simulink library "MBDS_Subsystems"  (R2018b)
settings: Solver=ode45  StartTime=0.0  StopTime=10.0  RelTol=1e-3
libraries: KIBES_Signal x1429, MBDS_Modules x44, simulink x2
(part 15 of 15)

== system MBDS_Subsystems/SUB_IoControl/PowerGroups ==
  bo_SendEnable : Inport
  in_DIAG_AnalogInputsPWR.IN_PWR_DIAG : KIBES_Signal/KIBES_Signal  MBDS_LibraryBlock=on  DatabaseKey=722  SignalName=DIAG_AnalogInputsPWR.IN_PWR_DIAG  SymbolName=DIAG_AnalogInputsPWR_IN_PWR_DIAG_000722  DataType=uint16  Init=1  Slope=1  Bias=0  DataSize=1  fpDataType=uint16  BlockIOType=Inport  DeviceType=0
  in_DIAG_AnalogInputsPWR.IN_PWR_G1_DIAG : KIBES_Signal/KIBES_Signal  MBDS_LibraryBlock=on  DatabaseKey=724  SignalName=DIAG_AnalogInputsPWR.IN_PWR_G1_DIAG  SymbolName=DIAG_AnalogInputsPWR_IN_PWR_G1_DIAG_000724  DataType=uint16  Init=1  Slope=1  Bias=0  DataSize=1  fpDataType=uint16  BlockIOType=Inport  DeviceType=0
  in_DIAG_AnalogInputsPWR.IN_PWR_G2_DIAG : KIBES_Signal/KIBES_Signal  MBDS_LibraryBlock=on  DatabaseKey=726  SignalName=DIAG_AnalogInputsPWR.IN_PWR_G2_DIAG  SymbolName=DIAG_AnalogInputsPWR_IN_PWR_G2_DIAG_000726  DataType=uint16  Init=1  Slope=1  Bias=0  DataSize=1  fpDataType=uint16  BlockIOType=Inport  DeviceType=0
  in_DIAG_AnalogInputsPWR.IN_PWR_G3_DIAG : KIBES_Signal/KIBES_Signal  MBDS_LibraryBlock=on  DatabaseKey=734  SignalName=DIAG_AnalogInputsPWR.IN_PWR_G3_DIAG  SymbolName=DIAG_AnalogInputsPWR_IN_PWR_G3_DIAG_000734  DataType=uint16  Init=1  Slope=1  Bias=0  DataSize=1  fpDataType=uint16  BlockIOType=Inport  DeviceType=0
  in_DIAG_AnalogInputsPWR.IN_PWR_G4_DIAG : KIBES_Signal/KIBES_Signal  MBDS_LibraryBlock=on  DatabaseKey=728  SignalName=DIAG_AnalogInputsPWR.IN_PWR_G4_DIAG  SymbolName=DIAG_AnalogInputsPWR_IN_PWR_G4_DIAG_000728  DataType=uint16  Init=1  Slope=1  Bias=0  DataSize=1  fpDataType=uint16  BlockIOType=Inport  DeviceType=0
  in_DIAG_AnalogInputsPWR.IN_PWR_G5_DIAG : KIBES_Signal/KIBES_Signal  MBDS_LibraryBlock=on  DatabaseKey=730  SignalName=DIAG_AnalogInputsPWR.IN_PWR_G5_DIAG  SymbolName=DIAG_AnalogInputsPWR_IN_PWR_G5_DIAG_000730  DataType=uint16  Init=1  Slope=1  Bias=0  DataSize=1  fpDataType=uint16  BlockIOType=Inport  DeviceType=0
  in_DIAG_AnalogInputsPWR.IN_PWR_G7_DIAG : KIBES_Signal/KIBES_Signal  MBDS_LibraryBlock=on  DatabaseKey=732  SignalName=DIAG_AnalogInputsPWR.IN_PWR_G7_DIAG  SymbolName=DIAG_AnalogInputsPWR_IN_PWR_G7_DIAG_000732  DataType=uint16  Init=1  Slope=1  Bias=0  DataSize=1  fpDataType=uint16  BlockIOType=Inport  DeviceType=0
  in_IN_AnalogInputsPWR.IN_PWR : KIBES_Signal/KIBES_Signal  MBDS_LibraryBlock=on  DatabaseKey=721  SignalName=IN_AnalogInputsPWR.IN_PWR  SymbolName=IN_AnalogInputsPWR_IN_PWR_000721  DataType=uint32  Init=0  Slope=1  Bias=0  DataSize=1  fpDataType=uint32  BlockIOType=Inport  DeviceType=0
  in_IN_AnalogInputsPWR.IN_PWR_G1 : KIBES_Signal/KIBES_Signal  MBDS_LibraryBlock=on  DatabaseKey=723  SignalName=IN_AnalogInputsPWR.IN_PWR_G1  SymbolName=IN_AnalogInputsPWR_IN_PWR_G1_000723  DataType=uint16  Init=0  Slope=1  Bias=0  DataSize=1  fpDataType=uint16  BlockIOType=Inport  DeviceType=0
  in_IN_AnalogInputsPWR.IN_PWR_G2 : KIBES_Signal/KIBES_Signal  MBDS_LibraryBlock=on  DatabaseKey=725  SignalName=IN_AnalogInputsPWR.IN_PWR_G2  SymbolName=IN_AnalogInputsPWR_IN_PWR_G2_000725  DataType=uint16  Init=0  Slope=1  Bias=0  DataSize=1  fpDataType=uint16  BlockIOType=Inport  DeviceType=0
  in_IN_AnalogInputsPWR.IN_PWR_G3 : KIBES_Signal/KIBES_Signal  MBDS_LibraryBlock=on  DatabaseKey=733  SignalName=IN_AnalogInputsPWR.IN_PWR_G3  SymbolName=IN_AnalogInputsPWR_IN_PWR_G3_000733  DataType=uint16  Init=0  Slope=1  Bias=0  DataSize=1  fpDataType=uint16  BlockIOType=Inport  DeviceType=0
  in_IN_AnalogInputsPWR.IN_PWR_G4 : KIBES_Signal/KIBES_Signal  MBDS_LibraryBlock=on  DatabaseKey=727  SignalName=IN_AnalogInputsPWR.IN_PWR_G4  SymbolName=IN_AnalogInputsPWR_IN_PWR_G4_000727  DataType=uint16  Init=0  Slope=1  Bias=0  DataSize=1  fpDataType=uint16  BlockIOType=Inport  DeviceType=0
  in_IN_AnalogInputsPWR.IN_PWR_G5 : KIBES_Signal/KIBES_Signal  MBDS_LibraryBlock=on  DatabaseKey=729  SignalName=IN_AnalogInputsPWR.IN_PWR_G5  SymbolName=IN_AnalogInputsPWR_IN_PWR_G5_000729  DataType=uint16  Init=0  Slope=1  Bias=0  DataSize=1  fpDataType=uint16  BlockIOType=Inport  DeviceType=0
  in_IN_AnalogInputsPWR.IN_PWR_G7 : KIBES_Signal/KIBES_Signal  MBDS_LibraryBlock=on  DatabaseKey=731  SignalName=IN_AnalogInputsPWR.IN_PWR_G7  SymbolName=IN_AnalogInputsPWR_IN_PWR_G7_000731  DataType=uint16  Init=0  Slope=1  Bias=0  DataSize=1  fpDataType=uint16  BlockIOType=Inport  DeviceType=0
  out_OUT_PCAN.Tx_Pwr.PWR_G1_Sts.MessageEnable : KIBES_Signal/KIBES_Signal  MBDS_LibraryBlock=on  DatabaseKey=1777  SignalName=OUT_PCAN.Tx_Pwr.PWR_G1_Sts.MessageEnable  SymbolName=OUT_PCAN_Tx_Pwr_PWR_G1_Sts_MessageEnable_001777  DataType=boolean  Init=0  Slope=1  Bias=0  DataSize=1  fpDataType=boolean  BlockIOType=Outport  DeviceType=0
  out_OUT_PCAN.Tx_Pwr.PWR_G1_Sts.PWR_Gx_DIAG : KIBES_Signal/KIBES_Signal  MBDS_LibraryBlock=on  DatabaseKey=1763  SignalName=OUT_PCAN.Tx_Pwr.PWR_G1_Sts.PWR_Gx_DIAG  SymbolName=OUT_PCAN_Tx_Pwr_PWR_G1_Sts_PWR_Gx_DIAG_001763  DataType=uint16  Init=0  Slope=1  Bias=0  DataSize=1  fpDataType=uint16  BlockIOType=Outport  DeviceType=0
  out_OUT_PCAN.Tx_Pwr.PWR_G1_Sts.PWR_Gx_Val : KIBES_Signal/KIBES_Signal  MBDS_LibraryBlock=on  DatabaseKey=1764  SignalName=OUT_PCAN.Tx_Pwr.PWR_G1_Sts.PWR_Gx_Val  SymbolName=OUT_PCAN_Tx_Pwr_PWR_G1_Sts_PWR_Gx_Val_001764  DataType=uint16  Init=0  Slope=1  Bias=0  DataSize=1  fpDataType=uint16  BlockIOType=Outport  DeviceType=0
  out_OUT_PCAN.Tx_Pwr.PWR_G2_Sts.MessageEnable : KIBES_Signal/KIBES_Signal  MBDS_LibraryBlock=on  DatabaseKey=1778  SignalName=OUT_PCAN.Tx_Pwr.PWR_G2_Sts.MessageEnable  SymbolName=OUT_PCAN_Tx_Pwr_PWR_G2_Sts_MessageEnable_001778  DataType=boolean  Init=0  Slope=1  Bias=0  DataSize=1  fpDataType=boolean  BlockIOType=Outport  DeviceType=0
  out_OUT_PCAN.Tx_Pwr.PWR_G2_Sts.PWR_Gx_DIAG : KIBES_Signal/KIBES_Signal  MBDS_LibraryBlock=on  DatabaseKey=1765  SignalName=OUT_PCAN.Tx_Pwr.PWR_G2_Sts.PWR_Gx_DIAG  SymbolName=OUT_PCAN_Tx_Pwr_PWR_G2_Sts_PWR_Gx_DIAG_001765  DataType=uint16  Init=0  Slope=1  Bias=0  DataSize=1  fpDataType=uint16  BlockIOType=Outport  DeviceType=0
  out_OUT_PCAN.Tx_Pwr.PWR_G2_Sts.PWR_Gx_Val : KIBES_Signal/KIBES_Signal  MBDS_LibraryBlock=on  DatabaseKey=1766  SignalName=OUT_PCAN.Tx_Pwr.PWR_G2_Sts.PWR_Gx_Val  SymbolName=OUT_PCAN_Tx_Pwr_PWR_G2_Sts_PWR_Gx_Val_001766  DataType=uint16  Init=0  Slope=1  Bias=0  DataSize=1  fpDataType=uint16  BlockIOType=Outport  DeviceType=0
  out_OUT_PCAN.Tx_Pwr.PWR_G3_Sts.MessageEnable : KIBES_Signal/KIBES_Signal  MBDS_LibraryBlock=on  DatabaseKey=1779  SignalName=OUT_PCAN.Tx_Pwr.PWR_G3_Sts.MessageEnable  SymbolName=OUT_PCAN_Tx_Pwr_PWR_G3_Sts_MessageEnable_001779  DataType=boolean  Init=0  Slope=1  Bias=0  DataSize=1  fpDataType=boolean  BlockIOType=Outport  DeviceType=0
  out_OUT_PCAN.Tx_Pwr.PWR_G3_Sts.PWR_Gx_DIAG : KIBES_Signal/KIBES_Signal  MBDS_LibraryBlock=on  DatabaseKey=1767  SignalName=OUT_PCAN.Tx_Pwr.PWR_G3_Sts.PWR_Gx_DIAG  SymbolName=OUT_PCAN_Tx_Pwr_PWR_G3_Sts_PWR_Gx_DIAG_001767  DataType=uint16  Init=0  Slope=1  Bias=0  DataSize=1  fpDataType=uint16  BlockIOType=Outport  DeviceType=0
  out_OUT_PCAN.Tx_Pwr.PWR_G3_Sts.PWR_Gx_Val : KIBES_Signal/KIBES_Signal  MBDS_LibraryBlock=on  DatabaseKey=1768  SignalName=OUT_PCAN.Tx_Pwr.PWR_G3_Sts.PWR_Gx_Val  SymbolName=OUT_PCAN_Tx_Pwr_PWR_G3_Sts_PWR_Gx_Val_001768  DataType=uint16  Init=0  Slope=1  Bias=0  DataSize=1  fpDataType=uint16  BlockIOType=Outport  DeviceType=0
  out_OUT_PCAN.Tx_Pwr.PWR_G4_Sts.MessageEnable : KIBES_Signal/KIBES_Signal  MBDS_LibraryBlock=on  DatabaseKey=1780  SignalName=OUT_PCAN.Tx_Pwr.PWR_G4_Sts.MessageEnable  SymbolName=OUT_PCAN_Tx_Pwr_PWR_G4_Sts_MessageEnable_001780  DataType=boolean  Init=0  Slope=1  Bias=0  DataSize=1  fpDataType=boolean  BlockIOType=Outport  DeviceType=0
  out_OUT_PCAN.Tx_Pwr.PWR_G4_Sts.PWR_Gx_DIAG : KIBES_Signal/KIBES_Signal  MBDS_LibraryBlock=on  DatabaseKey=1769  SignalName=OUT_PCAN.Tx_Pwr.PWR_G4_Sts.PWR_Gx_DIAG  SymbolName=OUT_PCAN_Tx_Pwr_PWR_G4_Sts_PWR_Gx_DIAG_001769  DataType=uint16  Init=0  Slope=1  Bias=0  DataSize=1  fpDataType=uint16  BlockIOType=Outport  DeviceType=0
  out_OUT_PCAN.Tx_Pwr.PWR_G4_Sts.PWR_Gx_Val : KIBES_Signal/KIBES_Signal  MBDS_LibraryBlock=on  DatabaseKey=1770  SignalName=OUT_PCAN.Tx_Pwr.PWR_G4_Sts.PWR_Gx_Val  SymbolName=OUT_PCAN_Tx_Pwr_PWR_G4_Sts_PWR_Gx_Val_001770  DataType=uint16  Init=0  Slope=1  Bias=0  DataSize=1  fpDataType=uint16  BlockIOType=Outport  DeviceType=0
  out_OUT_PCAN.Tx_Pwr.PWR_G5_Sts.MessageEnable : KIBES_Signal/KIBES_Signal  MBDS_LibraryBlock=on  DatabaseKey=1781  SignalName=OUT_PCAN.Tx_Pwr.PWR_G5_Sts.MessageEnable  SymbolName=OUT_PCAN_Tx_Pwr_PWR_G5_Sts_MessageEnable_001781  DataType=boolean  Init=0  Slope=1  Bias=0  DataSize=1  fpDataType=boolean  BlockIOType=Outport  DeviceType=0
  out_OUT_PCAN.Tx_Pwr.PWR_G5_Sts.PWR_Gx_DIAG : KIBES_Signal/KIBES_Signal  MBDS_LibraryBlock=on  DatabaseKey=1771  SignalName=OUT_PCAN.Tx_Pwr.PWR_G5_Sts.PWR_Gx_DIAG  SymbolName=OUT_PCAN_Tx_Pwr_PWR_G5_Sts_PWR_Gx_DIAG_001771  DataType=uint16  Init=0  Slope=1  Bias=0  DataSize=1  fpDataType=uint16  BlockIOType=Outport  DeviceType=0
  out_OUT_PCAN.Tx_Pwr.PWR_G5_Sts.PWR_Gx_Val : KIBES_Signal/KIBES_Signal  MBDS_LibraryBlock=on  DatabaseKey=1772  SignalName=OUT_PCAN.Tx_Pwr.PWR_G5_Sts.PWR_Gx_Val  SymbolName=OUT_PCAN_Tx_Pwr_PWR_G5_Sts_PWR_Gx_Val_001772  DataType=uint16  Init=0  Slope=1  Bias=0  DataSize=1  fpDataType=uint16  BlockIOType=Outport  DeviceType=0
  out_OUT_PCAN.Tx_Pwr.PWR_G7_Sts.MessageEnable : KIBES_Signal/KIBES_Signal  MBDS_LibraryBlock=on  DatabaseKey=1782  SignalName=OUT_PCAN.Tx_Pwr.PWR_G7_Sts.MessageEnable  SymbolName=OUT_PCAN_Tx_Pwr_PWR_G7_Sts_MessageEnable_001782  DataType=boolean  Init=0  Slope=1  Bias=0  DataSize=1  fpDataType=boolean  BlockIOType=Outport  DeviceType=0
  out_OUT_PCAN.Tx_Pwr.PWR_G7_Sts.PWR_Gx_DIAG : KIBES_Signal/KIBES_Signal  MBDS_LibraryBlock=on  DatabaseKey=1773  SignalName=OUT_PCAN.Tx_Pwr.PWR_G7_Sts.PWR_Gx_DIAG  SymbolName=OUT_PCAN_Tx_Pwr_PWR_G7_Sts_PWR_Gx_DIAG_001773  DataType=uint16  Init=0  Slope=1  Bias=0  DataSize=1  fpDataType=uint16  BlockIOType=Outport  DeviceType=0
  out_OUT_PCAN.Tx_Pwr.PWR_G7_Sts.PWR_Gx_Val : KIBES_Signal/KIBES_Signal  MBDS_LibraryBlock=on  DatabaseKey=1774  SignalName=OUT_PCAN.Tx_Pwr.PWR_G7_Sts.PWR_Gx_Val  SymbolName=OUT_PCAN_Tx_Pwr_PWR_G7_Sts_PWR_Gx_Val_001774  DataType=uint16  Init=0  Slope=1  Bias=0  DataSize=1  fpDataType=uint16  BlockIOType=Outport  DeviceType=0
  out_OUT_PCAN.Tx_Pwr.PWR_Sts.MessageEnable : KIBES_Signal/KIBES_Signal  MBDS_LibraryBlock=on  DatabaseKey=1783  SignalName=OUT_PCAN.Tx_Pwr.PWR_Sts.MessageEnable  SymbolName=OUT_PCAN_Tx_Pwr_PWR_Sts_MessageEnable_001783  DataType=boolean  Init=0  Slope=1  Bias=0  DataSize=1  fpDataType=boolean  BlockIOType=Outport  DeviceType=0
  out_OUT_PCAN.Tx_Pwr.PWR_Sts.PWR_DIAG : KIBES_Signal/KIBES_Signal  MBDS_LibraryBlock=on  DatabaseKey=1775  SignalName=OUT_PCAN.Tx_Pwr.PWR_Sts.PWR_DIAG  SymbolName=OUT_PCAN_Tx_Pwr_PWR_Sts_PWR_DIAG_001775  DataType=uint16  Init=0  Slope=1  Bias=0  DataSize=1  fpDataType=uint16  BlockIOType=Outport  DeviceType=0
  out_OUT_PCAN.Tx_Pwr.PWR_Sts.PWR_Val : KIBES_Signal/KIBES_Signal  MBDS_LibraryBlock=on  DatabaseKey=1776  SignalName=OUT_PCAN.Tx_Pwr.PWR_Sts.PWR_Val  SymbolName=OUT_PCAN_Tx_Pwr_PWR_Sts_PWR_Val_001776  DataType=uint32  Init=0  Slope=1  Bias=0  DataSize=1  fpDataType=uint32  BlockIOType=Outport  DeviceType=0
  wires:
  in_DIAG_AnalogInputsPWR.IN_PWR_G3_DIAG/1 -> out_OUT_PCAN.Tx_Pwr.PWR_G3_Sts.PWR_Gx_DIAG/1
  in_DIAG_AnalogInputsPWR.IN_PWR_G4_DIAG/1 -> out_OUT_PCAN.Tx_Pwr.PWR_G4_Sts.PWR_Gx_DIAG/1
  in_IN_AnalogInputsPWR.IN_PWR_G7/1 -> out_OUT_PCAN.Tx_Pwr.PWR_G7_Sts.PWR_Gx_Val/1
  in_IN_AnalogInputsPWR.IN_PWR_G3/1 -> out_OUT_PCAN.Tx_Pwr.PWR_G3_Sts.PWR_Gx_Val/1
  in_DIAG_AnalogInputsPWR.IN_PWR_G7_DIAG/1 -> out_OUT_PCAN.Tx_Pwr.PWR_G7_Sts.PWR_Gx_DIAG/1
  in_DIAG_AnalogInputsPWR.IN_PWR_G5_DIAG/1 -> out_OUT_PCAN.Tx_Pwr.PWR_G5_Sts.PWR_Gx_DIAG/1
  in_DIAG_AnalogInputsPWR.IN_PWR_G2_DIAG/1 -> out_OUT_PCAN.Tx_Pwr.PWR_G2_Sts.PWR_Gx_DIAG/1
  in_IN_AnalogInputsPWR.IN_PWR/1 -> out_OUT_PCAN.Tx_Pwr.PWR_Sts.PWR_Val/1
  in_DIAG_AnalogInputsPWR.IN_PWR_DIAG/1 -> out_OUT_PCAN.Tx_Pwr.PWR_Sts.PWR_DIAG/1
  in_DIAG_AnalogInputsPWR.IN_PWR_G1_DIAG/1 -> out_OUT_PCAN.Tx_Pwr.PWR_G1_Sts.PWR_Gx_DIAG/1
  in_IN_AnalogInputsPWR.IN_PWR_G4/1 -> out_OUT_PCAN.Tx_Pwr.PWR_G4_Sts.PWR_Gx_Val/1
  bo_SendEnable/1 -> out_OUT_PCAN.Tx_Pwr.PWR_G7_Sts.MessageEnable/1, out_OUT_PCAN.Tx_Pwr.PWR_Sts.MessageEnable/1, out_OUT_PCAN.Tx_Pwr.PWR_G5_Sts.MessageEnable/1, out_OUT_PCAN.Tx_Pwr.PWR_G4_Sts.MessageEnable/1, out_OUT_PCAN.Tx_Pwr.PWR_G3_Sts.MessageEnable/1, out_OUT_PCAN.Tx_Pwr.PWR_G2_Sts.MessageEnable/1, out_OUT_PCAN.Tx_Pwr.PWR_G1_Sts.MessageEnable/1
  in_IN_AnalogInputsPWR.IN_PWR_G5/1 -> out_OUT_PCAN.Tx_Pwr.PWR_G5_Sts.PWR_Gx_Val/1
  in_IN_AnalogInputsPWR.IN_PWR_G1/1 -> out_OUT_PCAN.Tx_Pwr.PWR_G1_Sts.PWR_Gx_Val/1
  in_IN_AnalogInputsPWR.IN_PWR_G2/1 -> out_OUT_PCAN.Tx_Pwr.PWR_G2_Sts.PWR_Gx_Val/1

== system MBDS_Subsystems/SUB_LinControl/AND1 ==
  note: AND
  u1 : Inport
  DataType : DataTypeConversion
  Operator : simulink/Logic and Bit Operations/Bitwise Operator  logicop=AND  UseBitMask=on  BitMask='FF'  BitMaskRealWorld=Stored Integer
  y : Outport
  wires:
  DataType/1 -> y/1
  u1/1 -> Operator/1
  Operator/1 -> DataType/1

== system MBDS_Subsystems/SUB_LinControl/AND2 ==
  note: AND
  u1 : Inport
  DataType : DataTypeConversion
  Operator : simulink/Logic and Bit Operations/Bitwise Operator  logicop=AND  UseBitMask=on  BitMask='FF00'  BitMaskRealWorld=Stored Integer
  y : Outport
  wires:
  DataType/1 -> y/1
  u1/1 -> Operator/1
  Operator/1 -> DataType/1

== system MBDS_Subsystems/SUB_SystemStates/NOT ==
  note: NOT
  u1 : Inport  OutDataTypeStr=boolean
  DataType : DataTypeConversion  OutDataTypeStr=boolean
  Operator : Logic  Operator=NOT  Inputs=1  AllPortsSameDT=off  OutDataTypeStr=boolean
  y : Outport
  wires:
  DataType/1 -> y/1
  u1/1 -> Operator/1
  Operator/1 -> DataType/1

== system MBDS_Subsystems/SUB_SystemStates/OR ==
  note: OR
  u1 : Inport  OutDataTypeStr=boolean
  u2 : Inport  Port=2  OutDataTypeStr=boolean
  u3 : Inport  Port=3  OutDataTypeStr=boolean
  u4 : Inport  Port=4  OutDataTypeStr=boolean
  u5 : Inport  Port=5  OutDataTypeStr=boolean
  u6 : Inport  Port=6  OutDataTypeStr=boolean
  u7 : Inport  Port=7  OutDataTypeStr=boolean
  u8 : Inport  Port=8  OutDataTypeStr=boolean
  DataType : DataTypeConversion  OutDataTypeStr=boolean
  Operator : Logic  Operator=OR  Inputs=8  AllPortsSameDT=off  OutDataTypeStr=boolean
  y : Outport
  wires:
  u8/1 -> Operator/8
  u7/1 -> Operator/7
  u6/1 -> Operator/6
  u5/1 -> Operator/5
  u4/1 -> Operator/4
  u3/1 -> Operator/3
  DataType/1 -> y/1
  u2/1 -> Operator/2
  u1/1 -> Operator/1
  Operator/1 -> DataType/1

== system MBDS_Subsystems/SUB_ExpIOControl/Outputs/AND ==
  note: AND
  u1 : Inport  OutDataTypeStr=boolean
  u2 : Inport  Port=2  OutDataTypeStr=boolean
  DataType : DataTypeConversion  OutDataTypeStr=boolean
  Operator : Logic  AllPortsSameDT=off  OutDataTypeStr=boolean
  y : Outport
  wires:
  DataType/1 -> y/1
  u2/1 -> Operator/2
  u1/1 -> Operator/1
  Operator/1 -> DataType/1

== system MBDS_Subsystems/SUB_ExpIOControl/Outputs/AND1 ==
  note: AND
  u1 : Inport  OutDataTypeStr=boolean
  u2 : Inport  Port=2  OutDataTypeStr=boolean
  DataType : DataTypeConversion  OutDataTypeStr=boolean
  Operator : Logic  AllPortsSameDT=off  OutDataTypeStr=boolean
  y : Outport
  wires:
  DataType/1 -> y/1
  u2/1 -> Operator/2
  u1/1 -> Operator/1
  Operator/1 -> DataType/1

== system MBDS_Subsystems/SUB_ExpIOControl/Outputs/AND10 ==
  note: AND
  u1 : Inport  OutDataTypeStr=boolean
  u2 : Inport  Port=2  OutDataTypeStr=boolean
  DataType : DataTypeConversion  OutDataTypeStr=boolean
  Operator : Logic  AllPortsSameDT=off  OutDataTypeStr=boolean
  y : Outport
  wires:
  DataType/1 -> y/1
  u2/1 -> Operator/2
  u1/1 -> Operator/1
  Operator/1 -> DataType/1

== system MBDS_Subsystems/SUB_ExpIOControl/Outputs/AND11 ==
  note: AND
  u1 : Inport  OutDataTypeStr=boolean
  u2 : Inport  Port=2  OutDataTypeStr=boolean
  DataType : DataTypeConversion  OutDataTypeStr=boolean
  Operator : Logic  AllPortsSameDT=off  OutDataTypeStr=boolean
  y : Outport
  wires:
  DataType/1 -> y/1
  u2/1 -> Operator/2
  u1/1 -> Operator/1
  Operator/1 -> DataType/1

== system MBDS_Subsystems/SUB_ExpIOControl/Outputs/AND12 ==
  note: AND
  u1 : Inport  OutDataTypeStr=boolean
  u2 : Inport  Port=2  OutDataTypeStr=boolean
  DataType : DataTypeConversion  OutDataTypeStr=boolean
  Operator : Logic  AllPortsSameDT=off  OutDataTypeStr=boolean
  y : Outport
  wires:
  DataType/1 -> y/1
  u2/1 -> Operator/2
  u1/1 -> Operator/1
  Operator/1 -> DataType/1

== system MBDS_Subsystems/SUB_ExpIOControl/Outputs/AND13 ==
  note: AND
  u1 : Inport  OutDataTypeStr=boolean
  u2 : Inport  Port=2  OutDataTypeStr=boolean
  DataType : DataTypeConversion  OutDataTypeStr=boolean
  Operator : Logic  AllPortsSameDT=off  OutDataTypeStr=boolean
  y : Outport
  wires:
  DataType/1 -> y/1
  u2/1 -> Operator/2
  u1/1 -> Operator/1
  Operator/1 -> DataType/1

== system MBDS_Subsystems/SUB_ExpIOControl/Outputs/AND14 ==
  note: AND
  u1 : Inport  OutDataTypeStr=boolean
  u2 : Inport  Port=2  OutDataTypeStr=boolean
  DataType : DataTypeConversion  OutDataTypeStr=boolean
  Operator : Logic  AllPortsSameDT=off  OutDataTypeStr=boolean
  y : Outport
  wires:
  DataType/1 -> y/1
  u2/1 -> Operator/2
  u1/1 -> Operator/1
  Operator/1 -> DataType/1

== system MBDS_Subsystems/SUB_ExpIOControl/Outputs/AND15 ==
  note: AND
  u1 : Inport  OutDataTypeStr=boolean
  u2 : Inport  Port=2  OutDataTypeStr=boolean
  DataType : DataTypeConversion  OutDataTypeStr=boolean
  Operator : Logic  AllPortsSameDT=off  OutDataTypeStr=boolean
  y : Outport
  wires:
  DataType/1 -> y/1
  u2/1 -> Operator/2
  u1/1 -> Operator/1
  Operator/1 -> DataType/1

== system MBDS_Subsystems/SUB_ExpIOControl/Outputs/AND16 ==
  note: AND
  u1 : Inport  OutDataTypeStr=boolean
  u2 : Inport  Port=2  OutDataTypeStr=boolean
  DataType : DataTypeConversion  OutDataTypeStr=boolean
  Operator : Logic  AllPortsSameDT=off  OutDataTypeStr=boolean
  y : Outport
  wires:
  DataType/1 -> y/1
  u2/1 -> Operator/2
  u1/1 -> Operator/1
  Operator/1 -> DataType/1

== system MBDS_Subsystems/SUB_ExpIOControl/Outputs/AND17 ==
  note: AND
  u1 : Inport  OutDataTypeStr=boolean
  u2 : Inport  Port=2  OutDataTypeStr=boolean
  DataType : DataTypeConversion  OutDataTypeStr=boolean
  Operator : Logic  AllPortsSameDT=off  OutDataTypeStr=boolean
  y : Outport
  wires:
  DataType/1 -> y/1
  u2/1 -> Operator/2
  u1/1 -> Operator/1
  Operator/1 -> DataType/1

== system MBDS_Subsystems/SUB_ExpIOControl/Outputs/AND18 ==
  note: AND
  u1 : Inport  OutDataTypeStr=boolean
  u2 : Inport  Port=2  OutDataTypeStr=boolean
  DataType : DataTypeConversion  OutDataTypeStr=boolean
  Operator : Logic  AllPortsSameDT=off  OutDataTypeStr=boolean
  y : Outport
  wires:
  DataType/1 -> y/1
  u2/1 -> Operator/2
  u1/1 -> Operator/1
  Operator/1 -> DataType/1

== system MBDS_Subsystems/SUB_ExpIOControl/Outputs/AND19 ==
  note: AND
  u1 : Inport  OutDataTypeStr=boolean
  u2 : Inport  Port=2  OutDataTypeStr=boolean
  DataType : DataTypeConversion  OutDataTypeStr=boolean
  Operator : Logic  AllPortsSameDT=off  OutDataTypeStr=boolean
  y : Outport
  wires:
  DataType/1 -> y/1
  u2/1 -> Operator/2
  u1/1 -> Operator/1
  Operator/1 -> DataType/1

== system MBDS_Subsystems/SUB_ExpIOControl/Outputs/AND2 ==
  note: AND
  u1 : Inport  OutDataTypeStr=boolean
  u2 : Inport  Port=2  OutDataTypeStr=boolean
  DataType : DataTypeConversion  OutDataTypeStr=boolean
  Operator : Logic  AllPortsSameDT=off  OutDataTypeStr=boolean
  y : Outport
  wires:
  DataType/1 -> y/1
  u2/1 -> Operator/2
  u1/1 -> Operator/1
  Operator/1 -> DataType/1

== system MBDS_Subsystems/SUB_ExpIOControl/Outputs/AND20 ==
  note: AND
  u1 : Inport  OutDataTypeStr=boolean
  u2 : Inport  Port=2  OutDataTypeStr=boolean
  DataType : DataTypeConversion  OutDataTypeStr=boolean
  Operator : Logic  AllPortsSameDT=off  OutDataTypeStr=boolean
  y : Outport
  wires:
  DataType/1 -> y/1
  u2/1 -> Operator/2
  u1/1 -> Operator/1
  Operator/1 -> DataType/1

== system MBDS_Subsystems/SUB_ExpIOControl/Outputs/AND21 ==
  note: AND
  u1 : Inport  OutDataTypeStr=boolean
  u2 : Inport  Port=2  OutDataTypeStr=boolean
  DataType : DataTypeConversion  OutDataTypeStr=boolean
  Operator : Logic  AllPortsSameDT=off  OutDataTypeStr=boolean
  y : Outport
  wires:
  DataType/1 -> y/1
  u2/1 -> Operator/2
  u1/1 -> Operator/1
  Operator/1 -> DataType/1

== system MBDS_Subsystems/SUB_ExpIOControl/Outputs/AND22 ==
  note: AND
  u1 : Inport  OutDataTypeStr=boolean
  u2 : Inport  Port=2  OutDataTypeStr=boolean
  DataType : DataTypeConversion  OutDataTypeStr=boolean
  Operator : Logic  AllPortsSameDT=off  OutDataTypeStr=boolean
  y : Outport
  wires:
  DataType/1 -> y/1
  u2/1 -> Operator/2
  u1/1 -> Operator/1
  Operator/1 -> DataType/1

== system MBDS_Subsystems/SUB_ExpIOControl/Outputs/AND23 ==
  note: AND
  u1 : Inport  OutDataTypeStr=boolean
  u2 : Inport  Port=2  OutDataTypeStr=boolean
  DataType : DataTypeConversion  OutDataTypeStr=boolean
  Operator : Logic  AllPortsSameDT=off  OutDataTypeStr=boolean
  y : Outport
  wires:
  DataType/1 -> y/1
  u2/1 -> Operator/2
  u1/1 -> Operator/1
  Operator/1 -> DataType/1

== system MBDS_Subsystems/SUB_ExpIOControl/Outputs/AND24 ==
  note: AND
  u1 : Inport  OutDataTypeStr=boolean
  u2 : Inport  Port=2  OutDataTypeStr=boolean
  DataType : DataTypeConversion  OutDataTypeStr=boolean
  Operator : Logic  AllPortsSameDT=off  OutDataTypeStr=boolean
  y : Outport
  wires:
  DataType/1 -> y/1
  u2/1 -> Operator/2
  u1/1 -> Operator/1
  Operator/1 -> DataType/1

== system MBDS_Subsystems/SUB_ExpIOControl/Outputs/AND3 ==
  note: AND
  u1 : Inport  OutDataTypeStr=boolean
  u2 : Inport  Port=2  OutDataTypeStr=boolean
  DataType : DataTypeConversion  OutDataTypeStr=boolean
  Operator : Logic  AllPortsSameDT=off  OutDataTypeStr=boolean
  y : Outport
  wires:
  DataType/1 -> y/1
  u2/1 -> Operator/2
  u1/1 -> Operator/1
  Operator/1 -> DataType/1

== system MBDS_Subsystems/SUB_ExpIOControl/Outputs/AND4 ==
  note: AND
  u1 : Inport  OutDataTypeStr=boolean
  u2 : Inport  Port=2  OutDataTypeStr=boolean
  DataType : DataTypeConversion  OutDataTypeStr=boolean
  Operator : Logic  AllPortsSameDT=off  OutDataTypeStr=boolean
  y : Outport
  wires:
  DataType/1 -> y/1
  u2/1 -> Operator/2
  u1/1 -> Operator/1
  Operator/1 -> DataType/1

== system MBDS_Subsystems/SUB_ExpIOControl/Outputs/AND5 ==
  note: AND
  u1 : Inport  OutDataTypeStr=boolean
  u2 : Inport  Port=2  OutDataTypeStr=boolean
  DataType : DataTypeConversion  OutDataTypeStr=boolean
  Operator : Logic  AllPortsSameDT=off  OutDataTypeStr=boolean
  y : Outport
  wires:
  DataType/1 -> y/1
  u2/1 -> Operator/2
  u1/1 -> Operator/1
  Operator/1 -> DataType/1

== system MBDS_Subsystems/SUB_ExpIOControl/Outputs/AND6 ==
  note: AND
  u1 : Inport  OutDataTypeStr=boolean
  u2 : Inport  Port=2  OutDataTypeStr=boolean
  DataType : DataTypeConversion  OutDataTypeStr=boolean
  Operator : Logic  AllPortsSameDT=off  OutDataTypeStr=boolean
  y : Outport
  wires:
  DataType/1 -> y/1
  u2/1 -> Operator/2
  u1/1 -> Operator/1
  Operator/1 -> DataType/1

== system MBDS_Subsystems/SUB_ExpIOControl/Outputs/AND7 ==
  note: AND
  u1 : Inport  OutDataTypeStr=boolean
  u2 : Inport  Port=2  OutDataTypeStr=boolean
  DataType : DataTypeConversion  OutDataTypeStr=boolean
  Operator : Logic  AllPortsSameDT=off  OutDataTypeStr=boolean
  y : Outport
  wires:
  DataType/1 -> y/1
  u2/1 -> Operator/2
  u1/1 -> Operator/1
  Operator/1 -> DataType/1

== system MBDS_Subsystems/SUB_ExpIOControl/Outputs/AND8 ==
  note: AND
  u1 : Inport  OutDataTypeStr=boolean
  u2 : Inport  Port=2  OutDataTypeStr=boolean
  DataType : DataTypeConversion  OutDataTypeStr=boolean
  Operator : Logic  AllPortsSameDT=off  OutDataTypeStr=boolean
  y : Outport
  wires:
  DataType/1 -> y/1
  u2/1 -> Operator/2
  u1/1 -> Operator/1
  Operator/1 -> DataType/1

== system MBDS_Subsystems/SUB_ExpIOControl/Outputs/AND9 ==
  note: AND
  u1 : Inport  OutDataTypeStr=boolean
  u2 : Inport  Port=2  OutDataTypeStr=boolean
  DataType : DataTypeConversion  OutDataTypeStr=boolean
  Operator : Logic  AllPortsSameDT=off  OutDataTypeStr=boolean
  y : Outport
  wires:
  DataType/1 -> y/1
  u2/1 -> Operator/2
  u1/1 -> Operator/1
  Operator/1 -> DataType/1

== system MBDS_Subsystems/SUB_ExpIOControl/Outputs/EQ ==
  note: EQ
  u1 : Inport
  u2 : Inport  Port=2
  Operator : RelationalOperator  Operator===  OutDataTypeStr=boolean  RndMeth=Nearest  InputSameDT=on
  y : Outport
  wires:
  u2/1 -> Operator/2
  u1/1 -> Operator/1
  Operator/1 -> y/1

== system MBDS_Subsystems/SUB_ExpIOControl/Outputs/EQ1 ==
  note: EQ
  u1 : Inport
  u2 : Inport  Port=2
  Operator : RelationalOperator  Operator===  OutDataTypeStr=boolean  RndMeth=Nearest  InputSameDT=on
  y : Outport
  wires:
  u2/1 -> Operator/2
  u1/1 -> Operator/1
  Operator/1 -> y/1

== system MBDS_Subsystems/SUB_ExpIOControl/Outputs/EQ2 ==
  note: EQ
  u1 : Inport
  u2 : Inport  Port=2
  Operator : RelationalOperator  Operator===  OutDataTypeStr=boolean  RndMeth=Nearest  InputSameDT=on
  y : Outport
  wires:
  u2/1 -> Operator/2
  u1/1 -> Operator/1
  Operator/1 -> y/1

== system MBDS_Subsystems/SUB_ExpIOControl/PowerGroups/AND1 ==
  note: AND
  u1 : Inport  OutDataTypeStr=boolean
  u2 : Inport  Port=2  OutDataTypeStr=boolean
  DataType : DataTypeConversion  OutDataTypeStr=boolean
  Operator : Logic  AllPortsSameDT=off  OutDataTypeStr=boolean
  y : Outport
  wires:
  DataType/1 -> y/1
  u2/1 -> Operator/2
  u1/1 -> Operator/1
  Operator/1 -> DataType/1

== system MBDS_Subsystems/SUB_ExpIOControl/PowerGroups/EQ ==
  note: EQ
  u1 : Inport
  u2 : Inport  Port=2
  Operator : RelationalOperator  Operator===  OutDataTypeStr=boolean  RndMeth=Nearest  InputSameDT=on
  y : Outport
  wires:
  u2/1 -> Operator/2
  u1/1 -> Operator/1
  Operator/1 -> y/1

== system MBDS_Subsystems/SUB_IoControl/AnalogInputs/AND ==
  note: AND
  u1 : Inport  OutDataTypeStr=boolean
  u2 : Inport  Port=2  OutDataTypeStr=boolean
  DataType : DataTypeConversion  OutDataTypeStr=boolean
  Operator : Logic  AllPortsSameDT=off  OutDataTypeStr=boolean
  y : Outport
  wires:
  DataType/1 -> y/1
  u2/1 -> Operator/2
  u1/1 -> Operator/1
  Operator/1 -> DataType/1

== system MBDS_Subsystems/SUB_IoControl/AnalogInputs/AND1 ==
  note: AND
  u1 : Inport  OutDataTypeStr=boolean
  u2 : Inport  Port=2  OutDataTypeStr=boolean
  DataType : DataTypeConversion  OutDataTypeStr=boolean
  Operator : Logic  AllPortsSameDT=off  OutDataTypeStr=boolean
  y : Outport
  wires:
  DataType/1 -> y/1
  u2/1 -> Operator/2
  u1/1 -> Operator/1
  Operator/1 -> DataType/1

== system MBDS_Subsystems/SUB_IoControl/AnalogInputs/AND2 ==
  note: AND
  u1 : Inport  OutDataTypeStr=boolean
  u2 : Inport  Port=2  OutDataTypeStr=boolean
  DataType : DataTypeConversion  OutDataTypeStr=boolean
  Operator : Logic  AllPortsSameDT=off  OutDataTypeStr=boolean
  y : Outport
  wires:
  DataType/1 -> y/1
  u2/1 -> Operator/2
  u1/1 -> Operator/1
  Operator/1 -> DataType/1

== system MBDS_Subsystems/SUB_IoControl/AnalogInputs/AND3 ==
  note: AND
  u1 : Inport  OutDataTypeStr=boolean
  u2 : Inport  Port=2  OutDataTypeStr=boolean
  DataType : DataTypeConversion  OutDataTypeStr=boolean
  Operator : Logic  AllPortsSameDT=off  OutDataTypeStr=boolean
  y : Outport
  wires:
  DataType/1 -> y/1
  u2/1 -> Operator/2
  u1/1 -> Operator/1
  Operator/1 -> DataType/1

== system MBDS_Subsystems/SUB_IoControl/AnalogInputs/EQ ==
  note: EQ
  u1 : Inport
  u2 : Inport  Port=2
  Operator : RelationalOperator  Operator===  OutDataTypeStr=boolean  RndMeth=Nearest  InputSameDT=on
  y : Outport
  wires:
  u2/1 -> Operator/2
  u1/1 -> Operator/1
  Operator/1 -> y/1

== system MBDS_Subsystems/SUB_IoControl/AnalogsSupply/AND ==
  note: AND
  u1 : Inport  OutDataTypeStr=boolean
  u2 : Inport  Port=2  OutDataTypeStr=boolean
  DataType : DataTypeConversion  OutDataTypeStr=boolean
  Operator : Logic  AllPortsSameDT=off  OutDataTypeStr=boolean
  y : Outport
  wires:
  DataType/1 -> y/1
  u2/1 -> Operator/2
  u1/1 -> Operator/1
  Operator/1 -> DataType/1

== system MBDS_Subsystems/SUB_IoControl/AnalogsSupply/AND1 ==
  note: AND
  u1 : Inport  OutDataTypeStr=boolean
  u2 : Inport  Port=2  OutDataTypeStr=boolean
  DataType : DataTypeConversion  OutDataTypeStr=boolean
  Operator : Logic  AllPortsSameDT=off  OutDataTypeStr=boolean
  y : Outport
  wires:
  DataType/1 -> y/1
  u2/1 -> Operator/2
  u1/1 -> Operator/1
  Operator/1 -> DataType/1

== system MBDS_Subsystems/SUB_IoControl/AnalogsSupply/AND2 ==
  note: AND
  u1 : Inport  OutDataTypeStr=boolean
  u2 : Inport  Port=2  OutDataTypeStr=boolean
  DataType : DataTypeConversion  OutDataTypeStr=boolean
  Operator : Logic  AllPortsSameDT=off  OutDataTypeStr=boolean
  y : Outport
  wires:
  DataType/1 -> y/1
  u2/1 -> Operator/2
  u1/1 -> Operator/1
  Operator/1 -> DataType/1

== system MBDS_Subsystems/SUB_IoControl/AnalogsSupply/EQ ==
  note: EQ
  u1 : Inport
  u2 : Inport  Port=2
  Operator : RelationalOperator  Operator===  OutDataTypeStr=boolean  RndMeth=Nearest  InputSameDT=on
  y : Outport
  wires:
  u2/1 -> Operator/2
  u1/1 -> Operator/1
  Operator/1 -> y/1

== system MBDS_Subsystems/SUB_IoControl/DigitalOutputs/AND1 ==
  note: AND
  u1 : Inport  OutDataTypeStr=boolean
  u2 : Inport  Port=2  OutDataTypeStr=boolean
  DataType : DataTypeConversion  OutDataTypeStr=boolean
  Operator : Logic  AllPortsSameDT=off  OutDataTypeStr=boolean
  y : Outport
  wires:
  DataType/1 -> y/1
  u2/1 -> Operator/2
  u1/1 -> Operator/1
  Operator/1 -> DataType/1

== system MBDS_Subsystems/SUB_IoControl/DigitalOutputs/AND10 ==
  note: AND
  u1 : Inport  OutDataTypeStr=boolean
  u2 : Inport  Port=2  OutDataTypeStr=boolean
  DataType : DataTypeConversion  OutDataTypeStr=boolean
  Operator : Logic  AllPortsSameDT=off  OutDataTypeStr=boolean
  y : Outport
  wires:
  DataType/1 -> y/1
  u2/1 -> Operator/2
  u1/1 -> Operator/1
  Operator/1 -> DataType/1

== system MBDS_Subsystems/SUB_IoControl/DigitalOutputs/AND11 ==
  note: AND
  u1 : Inport  OutDataTypeStr=boolean
  u2 : Inport  Port=2  OutDataTypeStr=boolean
  DataType : DataTypeConversion  OutDataTypeStr=boolean
  Operator : Logic  AllPortsSameDT=off  OutDataTypeStr=boolean
  y : Outport
  wires:
  DataType/1 -> y/1
  u2/1 -> Operator/2
  u1/1 -> Operator/1
  Operator/1 -> DataType/1

== system MBDS_Subsystems/SUB_IoControl/DigitalOutputs/AND12 ==
  note: AND
  u1 : Inport  OutDataTypeStr=boolean
  u2 : Inport  Port=2  OutDataTypeStr=boolean
  DataType : DataTypeConversion  OutDataTypeStr=boolean
  Operator : Logic  AllPortsSameDT=off  OutDataTypeStr=boolean
  y : Outport
  wires:
  DataType/1 -> y/1
  u2/1 -> Operator/2
  u1/1 -> Operator/1
  Operator/1 -> DataType/1

== system MBDS_Subsystems/SUB_IoControl/DigitalOutputs/AND13 ==
  note: AND
  u1 : Inport  OutDataTypeStr=boolean
  u2 : Inport  Port=2  OutDataTypeStr=boolean
  DataType : DataTypeConversion  OutDataTypeStr=boolean
  Operator : Logic  AllPortsSameDT=off  OutDataTypeStr=boolean
  y : Outport
  wires:
  DataType/1 -> y/1
  u2/1 -> Operator/2
  u1/1 -> Operator/1
  Operator/1 -> DataType/1

== system MBDS_Subsystems/SUB_IoControl/DigitalOutputs/AND14 ==
  note: AND
  u1 : Inport  OutDataTypeStr=boolean
  u2 : Inport  Port=2  OutDataTypeStr=boolean
  DataType : DataTypeConversion  OutDataTypeStr=boolean
  Operator : Logic  AllPortsSameDT=off  OutDataTypeStr=boolean
  y : Outport
  wires:
  DataType/1 -> y/1
  u2/1 -> Operator/2
  u1/1 -> Operator/1
  Operator/1 -> DataType/1

== system MBDS_Subsystems/SUB_IoControl/DigitalOutputs/AND15 ==
  note: AND
  u1 : Inport  OutDataTypeStr=boolean
  u2 : Inport  Port=2  OutDataTypeStr=boolean
  DataType : DataTypeConversion  OutDataTypeStr=boolean
  Operator : Logic  AllPortsSameDT=off  OutDataTypeStr=boolean
  y : Outport
  wires:
  DataType/1 -> y/1
  u2/1 -> Operator/2
  u1/1 -> Operator/1
  Operator/1 -> DataType/1

== system MBDS_Subsystems/SUB_IoControl/DigitalOutputs/AND16 ==
  note: AND
  u1 : Inport  OutDataTypeStr=boolean
  u2 : Inport  Port=2  OutDataTypeStr=boolean
  DataType : DataTypeConversion  OutDataTypeStr=boolean
  Operator : Logic  AllPortsSameDT=off  OutDataTypeStr=boolean
  y : Outport
  wires:
  DataType/1 -> y/1
  u2/1 -> Operator/2
  u1/1 -> Operator/1
  Operator/1 -> DataType/1

== system MBDS_Subsystems/SUB_IoControl/DigitalOutputs/AND17 ==
  note: AND
  u1 : Inport  OutDataTypeStr=boolean
  u2 : Inport  Port=2  OutDataTypeStr=boolean
  DataType : DataTypeConversion  OutDataTypeStr=boolean
  Operator : Logic  AllPortsSameDT=off  OutDataTypeStr=boolean
  y : Outport
  wires:
  DataType/1 -> y/1
  u2/1 -> Operator/2
  u1/1 -> Operator/1
  Operator/1 -> DataType/1

== system MBDS_Subsystems/SUB_IoControl/DigitalOutputs/AND18 ==
  note: AND
  u1 : Inport  OutDataTypeStr=boolean
  u2 : Inport  Port=2  OutDataTypeStr=boolean
  DataType : DataTypeConversion  OutDataTypeStr=boolean
  Operator : Logic  AllPortsSameDT=off  OutDataTypeStr=boolean
  y : Outport
  wires:
  DataType/1 -> y/1
  u2/1 -> Operator/2
  u1/1 -> Operator/1
  Operator/1 -> DataType/1

== system MBDS_Subsystems/SUB_IoControl/DigitalOutputs/EQ ==
  note: EQ
  u1 : Inport
  u2 : Inport  Port=2
  Operator : RelationalOperator  Operator===  OutDataTypeStr=boolean  RndMeth=Nearest  InputSameDT=on
  y : Outport
  wires:
  u2/1 -> Operator/2
  u1/1 -> Operator/1
  Operator/1 -> y/1

== system MBDS_Subsystems/SUB_IoControl/PWMs/AND ==
  note: AND
  u1 : Inport  OutDataTypeStr=boolean
  u2 : Inport  Port=2  OutDataTypeStr=boolean
  DataType : DataTypeConversion  OutDataTypeStr=boolean
  Operator : Logic  AllPortsSameDT=off  OutDataTypeStr=boolean
  y : Outport
  wires:
  DataType/1 -> y/1
  u2/1 -> Operator/2
  u1/1 -> Operator/1
  Operator/1 -> DataType/1

== system MBDS_Subsystems/SUB_IoControl/PWMs/AND1 ==
  note: AND
  u1 : Inport  OutDataTypeStr=boolean
  u2 : Inport  Port=2  OutDataTypeStr=boolean
  DataType : DataTypeConversion  OutDataTypeStr=boolean
  Operator : Logic  AllPortsSameDT=off  OutDataTypeStr=boolean
  y : Outport
  wires:
  DataType/1 -> y/1
  u2/1 -> Operator/2
  u1/1 -> Operator/1
  Operator/1 -> DataType/1

== system MBDS_Subsystems/SUB_IoControl/PWMs/EQ ==
  note: EQ
  u1 : Inport
  u2 : Inport  Port=2
  Operator : RelationalOperator  Operator===  OutDataTypeStr=boolean  RndMeth=Nearest  InputSameDT=on
  y : Outport
  wires:
  u2/1 -> Operator/2
  u1/1 -> Operator/1
  Operator/1 -> y/1

== system MBDS_Subsystems/SUB_IoControl/PWMs/EQ1 ==
  note: EQ
  u1 : Inport
  u2 : Inport  Port=2
  Operator : RelationalOperator  Operator===  OutDataTypeStr=boolean  RndMeth=Nearest  InputSameDT=on
  y : Outport
  wires:
  u2/1 -> Operator/2
  u1/1 -> Operator/1
  Operator/1 -> y/1

== system MBDS_Subsystems/SUB_IoControl/PWMs/GT ==
  note: GT
  u1 : Inport
  u2 : Inport  Port=2
  Operator : RelationalOperator  Operator=>  OutDataTypeStr=boolean  RndMeth=Nearest  InputSameDT=on
  y : Outport
  wires:
  Operator/1 -> y/1
  u1/1 -> Operator/1
  u2/1 -> Operator/2

== system MBDS_Subsystems/SUB_IoControl/PWMs/GT1 ==
  note: GT
  u1 : Inport
  u2 : Inport  Port=2
  Operator : RelationalOperator  Operator=>  OutDataTypeStr=boolean  RndMeth=Nearest  InputSameDT=on
  y : Outport
  wires:
  Operator/1 -> y/1
  u1/1 -> Operator/1
  u2/1 -> Operator/2

== system MBDS_Subsystems/SUB_IoControl/PWMs/GT2 ==
  note: GT
  u1 : Inport
  u2 : Inport  Port=2
  Operator : RelationalOperator  Operator=>  OutDataTypeStr=boolean  RndMeth=Nearest  InputSameDT=on
  y : Outport
  wires:
  Operator/1 -> y/1
  u1/1 -> Operator/1
  u2/1 -> Operator/2

== system MBDS_Subsystems/SUB_IoControl/PWMs/GT3 ==
  note: GT
  u1 : Inport
  u2 : Inport  Port=2
  Operator : RelationalOperator  Operator=>  OutDataTypeStr=boolean  RndMeth=Nearest  InputSameDT=on
  y : Outport
  wires:
  Operator/1 -> y/1
  u1/1 -> Operator/1
  u2/1 -> Operator/2

== system MBDS_Subsystems/SUB_IoControl/PWMs/GT4 ==
  note: GT
  u1 : Inport
  u2 : Inport  Port=2
  Operator : RelationalOperator  Operator=>  OutDataTypeStr=boolean  RndMeth=Nearest  InputSameDT=on
  y : Outport
  wires:
  Operator/1 -> y/1
  u1/1 -> Operator/1
  u2/1 -> Operator/2

== system MBDS_Subsystems/SUB_IoControl/PWMs/GT5 ==
  note: GT
  u1 : Inport
  u2 : Inport  Port=2
  Operator : RelationalOperator  Operator=>  OutDataTypeStr=boolean  RndMeth=Nearest  InputSameDT=on
  y : Outport
  wires:
  Operator/1 -> y/1
  u1/1 -> Operator/1
  u2/1 -> Operator/2

== system MBDS_Subsystems/SUB_IoControl/PWMs/GT6 ==
  note: GT
  u1 : Inport
  u2 : Inport  Port=2
  Operator : RelationalOperator  Operator=>  OutDataTypeStr=boolean  RndMeth=Nearest  InputSameDT=on
  y : Outport
  wires:
  Operator/1 -> y/1
  u1/1 -> Operator/1
  u2/1 -> Operator/2

== system MBDS_Subsystems/SUB_IoControl/PWMs/GT7 ==
  note: GT
  u1 : Inport
  u2 : Inport  Port=2
  Operator : RelationalOperator  Operator=>  OutDataTypeStr=boolean  RndMeth=Nearest  InputSameDT=on
  y : Outport
  wires:
  Operator/1 -> y/1
  u1/1 -> Operator/1
  u2/1 -> Operator/2

== system MBDS_Subsystems/SUB_IoControl/PWMs/GT8 ==
  note: GT
  u1 : Inport
  u2 : Inport  Port=2
  Operator : RelationalOperator  Operator=>  OutDataTypeStr=boolean  RndMeth=Nearest  InputSameDT=on
  y : Outport
  wires:
  Operator/1 -> y/1
  u1/1 -> Operator/1
  u2/1 -> Operator/2

== stateflow chart MBDS_Subsystems/SUB_IoControl/DigitalOutputs/BlinkSource ==
  state Blink_ON
    en:
    u16_Timer=uint16(1);
    bo_Blink = true;
    du:
    u16_Timer++;
  state Blink_OFF
    en:
    u16_Timer=uint16(1);
    bo_Blink = false;
    du:
    u16_Timer++;
  (default) -> Blink_ON
  Blink_OFF -> Blink_ON : [u16_Timer >= u16_PeriodTime]
  Blink_ON -> Blink_OFF : [u16_Timer >= u16_PeriodTime]
  data: u16_Timer local uint16 =0; bo_Blink output boolean =false; u16_PeriodTime input uint16 =12

== stateflow chart MBDS_Subsystems/SUB_SystemStates/ModelHoldForceTrue ==
  state WakeUp_ModelHoldTrue
    en:
    u16_Timer=uint16(0);
    bo_ModelHold = true;
    du:
    u16_Timer++;
  state Release_ModelHoldTrue
    en:
    bo_ModelHold = false;
  (default) -> WakeUp_ModelHoldTrue
  WakeUp_ModelHoldTrue -> Release_ModelHoldTrue : [u16_Timer >= u16_WakeUpForceHoldTime]
  data: u16_Timer local uint16 =0; bo_ModelHold output boolean =false; u16_WakeUpForceHoldTime input uint16
